simulink model "dynamic_twotrack_model"  (R2019a)
settings: Solver=VariableStepAuto  StartTime=0.0  StopTime=100  RelTol=1e-3
values from neighbouring files (symbols this model uses):
  cornering_stiffness = 1000    [config_dynamic_twotrack_model.m]
  init_states = [0; 0; 0; 0; 0; 0]    [config_dynamic_twotrack_model.m]
  length_front = 1    [config_dynamic_twotrack_model.m]
  length_rear = 1    [config_dynamic_twotrack_model.m]
  length_width = 0.5    [config_dynamic_twotrack_model.m]
  mass = 200    [config_dynamic_twotrack_model.m]
  yaw_inertia = 1000    [config_dynamic_twotrack_model.m]
libraries: simulink_extras x1, simulink x1
settings Model: Creator=jacoboffersen  LastModifiedBy=jacoboffersen

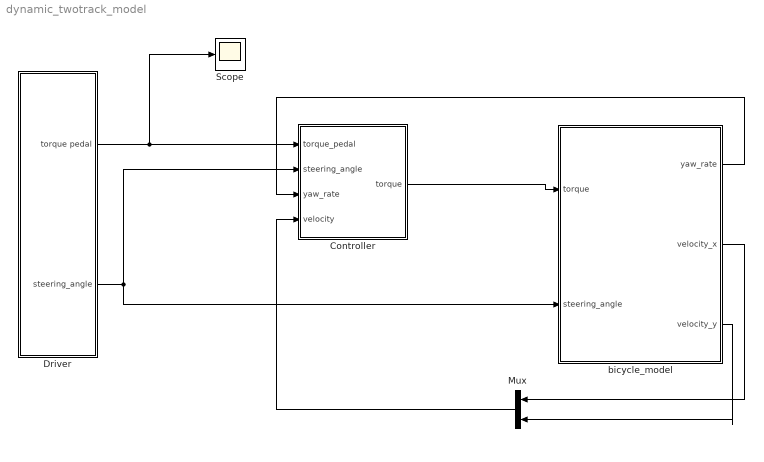
== system dynamic_twotrack_model ==
  Controller : Subsystem
  Driver : Subsystem
  Mux : Mux  Inputs=2
  Scope : Scope
  "bicycle_model " : Subsystem
  wires:
  Driver/2(steering_angle) -> "bicycle_model "/2("steering_angle "), Controller/2(steering_angle)
  Controller/1(torque) -> "bicycle_model "/1(torque)
  Driver/1(torque pedal) -> Scope/1, Controller/1(torque_pedal)
  Mux/1 -> Controller/4(velocity)
  "bicycle_model "/1(yaw_rate) -> Controller/3(yaw_rate)
  "bicycle_model "/2(velocity_x) -> Mux/1
  "bicycle_model "/3(velocity_y) -> Mux/2

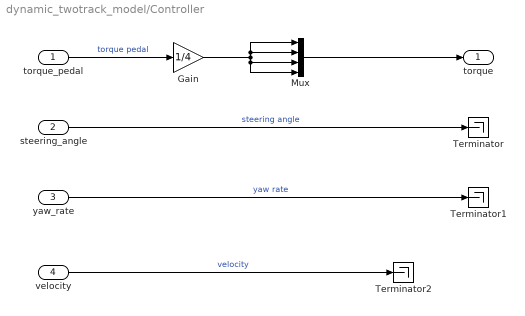
== system dynamic_twotrack_model/Controller ==
  torque_pedal : Inport
  steering_angle : Inport  Port=2
  yaw_rate : Inport  Port=3
  velocity : Inport  Port=4
  Gain : Gain  Gain=1/4
  Mux : Mux
  Terminator : Terminator
  Terminator1 : Terminator
  Terminator2 : Terminator
  torque : Outport
  wires:
  torque_pedal/1 -> Gain/1  "torque pedal"
  steering_angle/1 -> Terminator/1  "steering angle"
  yaw_rate/1 -> Terminator1/1  "yaw rate"
  velocity/1 -> Terminator2/1  "velocity"
  Mux/1 -> torque/1
  Gain/1 -> Mux/2, Mux/1, Mux/4, Mux/3

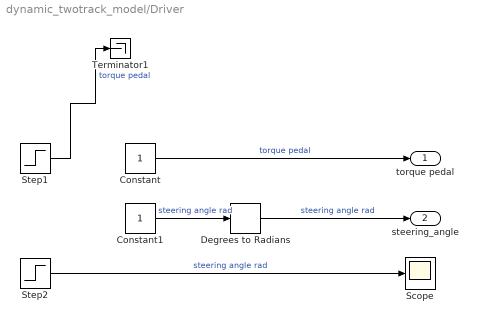
== system dynamic_twotrack_model/Driver ==
  Constant : Constant
  Constant1 : Constant
  Degrees to Radians : simulink_extras/Transformations/Degrees to Radians
  Scope : Scope
  Step1 : Step  Time=2  After=0  SampleTime=0
  Step2 : Step  Time=3  After=5  SampleTime=0
  Terminator1 : Terminator
  torque pedal : Outport
  steering_angle : Outport  Port=2
  wires:
  Constant/1 -> torque pedal/1  "torque pedal"
  Degrees to Radians/1 -> steering_angle/1  "steering angle rad"
  Step1/1 -> Terminator1/1  "torque pedal"
  Constant1/1 -> Degrees to Radians/1  "steering angle rad"
  Step2/1 -> Scope/1  "steering angle rad"

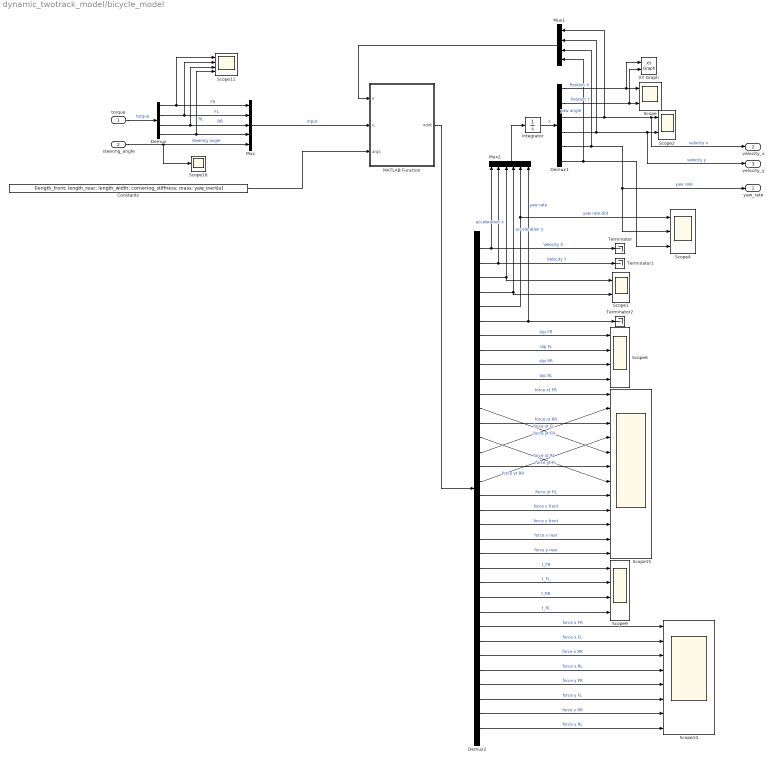
== system dynamic_twotrack_model/bicycle_model  ==
  torque : Inport
  "steering_angle " : Inport  Port=2
  Constants : Constant  Value=[length_front; length_rear; length_width; cornering_stiffness; mass; yaw_inertia]
  Demux : Demux
  Demux1 : Demux  Outputs=6
  Demux2 : Demux  Outputs=34
  Integrator : Integrator  InitialCondition=[init_states]
  MATLAB Function : MATLAB Function  TreatAsAtomicUnit=on
  Mux : Mux  Inputs=5
  Mux1 : Mux
  Mux2 : Mux  Inputs=6
  Scope : Scope  NumInputPorts=2
  Scope1 : Scope  NumInputPorts=2
  Scope10 : Scope
  Scope11 : Scope  NumInputPorts=4
  Scope14 : Scope  NumInputPorts=8
  Scope15 : Scope  NumInputPorts=12
  Scope2 : Scope  NumInputPorts=2
  Scope4 : Scope  NumInputPorts=3
  Scope6 : Scope  NumInputPorts=4
  Scope9 : Scope  NumInputPorts=4
  Terminator : Terminator
  Terminator1 : Terminator
  Terminator2 : Terminator
  XY Graph : simulink/Sinks/XY Graph  xmin=-10000  xmax=10000  ymin=-10000  ymax=10000  st=-1
  yaw_rate : Outport
  velocity_x : Outport  Port=2
  velocity_y : Outport  Port=3
  wires:
  Mux/1 -> MATLAB Function/2(u)  "input"
  "steering_angle "/1 -> Scope10/1, Mux/5  "steering angle"
  Constants/1 -> MATLAB Function/3(args)
  MATLAB Function/1(xdot) -> Demux2/1
  torque/1 -> Demux/1  "torque"
  Demux/4 -> Scope11/4, Mux/4  "RL"
  Demux/3 -> Scope11/3, Mux/3  "RR"
  Demux/2 -> Scope11/2, Mux/2  "FL"
  Demux/1 -> Scope11/1, Mux/1  "FR"
  Integrator/1 -> Demux1/1  "x"
  Mux1/1 -> MATLAB Function/1(x)
  Demux1/6 -> Scope4/3, Mux1/4  "yaw angle"
  Demux1/5 -> Mux1/3, Scope4/2, yaw_rate/1  "yaw rate"
  Demux1/4 -> velocity_y/1, Scope2/2, Mux1/2  "velocity y"
  Demux1/3 -> velocity_x/1, Scope2/1, Mux1/1  "velocity x"
  Demux2/1 -> Mux2/1, Terminator/1  "Velocity X"
  Demux2/2 -> Mux2/2, Terminator1/1  "Velocity Y"
  Demux2/3 -> Mux2/3, Scope1/1  "acceleration x"
  Demux2/4 -> Mux2/4, Scope1/2  "acceleration y"
  Demux2/5 -> Mux2/5, Scope4/1  "yaw rate dot"
  Demux2/6 -> Mux2/6, Terminator2/1  "yaw rate"
  Demux1/1 -> XY Graph/1, Scope/1  "Position X"
  Demux1/2 -> XY Graph/2, Scope/2  "Position Y"
  Mux2/1 -> Integrator/1
  Demux2/7 -> Scope6/1  "slip FR"
  Demux2/8 -> Scope6/2  "slip FL"
  Demux2/9 -> Scope6/3  "slip RR"
  Demux2/10 -> Scope6/4  "slip RL"
  Demux2/14 -> Scope15/7  "force xt RL"
  Demux2/13 -> Scope15/3  "force xt RR"
  Demux2/12 -> Scope15/5  "force xt FL"
  Demux2/11 -> Scope15/1  "force xt FR"
  Demux2/15 -> Scope15/2  "force yt FR"
  Demux2/16 -> Scope15/6  "force yt FL"
  Demux2/17 -> Scope15/4  "force yt RR"
  Demux2/18 -> Scope15/8  "force yt RL"
  Demux2/23 -> Scope9/1  "t_FR"
  Demux2/24 -> Scope9/2  "t_FL"
  Demux2/25 -> Scope9/3  "t_RR"
  Demux2/26 -> Scope9/4  "t_RL"
  Demux2/19 -> Scope15/9  "force x front"
  Demux2/20 -> Scope15/10  "force y front"
  Demux2/21 -> Scope15/11  "force x rear"
  Demux2/22 -> Scope15/12  "force y rear"
  Demux2/27 -> Scope14/1  "force x FR"
  Demux2/28 -> Scope14/2  "force x FL"
  Demux2/29 -> Scope14/3  "force x RR"
  Demux2/30 -> Scope14/4  "force x RL"
  Demux2/31 -> Scope14/5  "force y FR"
  Demux2/32 -> Scope14/6  "force y FL"
  Demux2/33 -> Scope14/7  "force y RR"
  Demux2/34 -> Scope14/8  "force y RL"

== matlab function dynamic_twotrack_model/bicycle_model /MATLAB Function ==
  data: x input; xdot output; u input; args input
function xdot = fcn(x, u, args)

% States
velocity_x       = x(1); 
velocity_y       = x(2); 
yaw_rate         = x(3); 
yaw_angle        = x(4); 

% System inputs
torque_FR        = u(1); 
torque_FL        = u(2); 
torque_RR        = u(3); 
torque_RL        = u(4); 
steering_angle   = u(5); 

% Constants
length_front        = args(1); 
length_rear         = args(2); 
length_width        = args(3); 
cornering_stiffness = args(4);
mass                = args(5);
yaw_inertia         = args(6);

g = 9.82;


Velocity_X = velocity_x * cos(yaw_angle) - velocity_y*sin(yaw_angle);
Velocity_Y = velocity_x * sin(yaw_angle) + velocity_y*cos(yaw_angle);


% Load transfer
lt_FR = 0;
lt_FL = 0;
lt_RR = 0;
lt_RL = 0;





% Vertical force on each wheel
force_z_FR = mass * g/4 + lt_FR;
force_z_FL = mass * g/4 + lt_FL;
force_z_RR = mass * g/4 + lt_RR;
force_z_RL = mass * g/4 + lt_RL;

% Longitudinal force on each wheel
force_x_factor = 1;
force_x_FR = torque_FR * force_z_FR * force_x_factor;
force_x_FL = torque_FL * force_z_FL * force_x_factor;
force_x_RR = torque_RR * force_z_RR * force_x_factor;
force_x_RL = torque_RL * force_z_RL * force_x_factor;


% Slip for each wheel
slip_FR = 0;
slip_FL = 0;
slip_RR = 0;
slip_RL = 0;
t_FR = 0;
t_FL = 0;
t_RR = 0;
t_RL = 0;
if velocity_x ~= 0 %&& yaw_rate ~= 0
%     slip_FR = steering_angle - atan((velocity_y+length_front*yaw_rate)/...
%                                     min(100000, velocity_x+length_width*yaw_rate));
% 
%     slip_FL = steering_angle - atan((velocity_y+length_front*yaw_rate)/...
%                                     min(100000, velocity_x-length_width*yaw_rate));
% 
%     slip_RR = - atan((velocity_y+length_rear*yaw_rate)/...
%                      min(100000, velocity_x+length_width*yaw_rate));
% 
%     slip_RL = - atan((velocity_y+length_rear*yaw_rate)/...
%                      min(100000, velocity_x-length_width*yaw_rate));
%     t_FR = - atan((velocity_y+length_front*yaw_rate)/...
%                   min(100000, velocity_x+length_width*yaw_rate));
%     t_FL = - atan((velocity_y+length_front*yaw_rate)/...
%                   min(100000, velocity_x-length_width*yaw_rate));
%     t_RR = - atan((velocity_y+length_rear*yaw_rate)/...
%                   min(100000, velocity_x+length_width*yaw_rate));
%     t_RL = - atan((velocity_y+length_rear*yaw_rate)/...
%                   min(100000, velocity_x-length_width*yaw_rate));
end
% 
slip_FR =   steering_angle * velocity_x * 0.1;
slip_FL =   steering_angle * velocity_x * 0.1;
slip_RR = - steering_angle * velocity_x * 0.05;
slip_RL = - steering_angle * velocity_x * 0.05;


% if velocity_x ~= 0 %&& yaw_rate ~= 0
%     beta = atan(length_rear/(length_front+length_rear)*tan(steering_angle));
%     slip_FR = steering_angle - beta - 1/velocity_x*(length_front/length_width)*yaw_rate;
%     slip_FL = steering_angle - beta - 1/velocity_x*(length_front/(length_width))*yaw_rate;
%     slip_RR = - atan((velocity_y+length_rear*yaw_rate)/...
%                      (velocity_x+length_width*yaw_rate));
% 
%     slip_RL = - atan((velocity_y+length_rear*yaw_rate)/...
%                      (velocity_x-length_width*yaw_rate));
% end

% Lateral force on each wheel
force_y_FR = cornering_stiffness * slip_FR;
force_y_FL = cornering_stiffness * slip_FL;
force_y_RR = cornering_stiffness * slip_RR;
force_y_RL = cornering_stiffness * slip_RL;

% Each force composant on each wheel
% FR
F_xx_FR = force_x_FR*cos(steering_angle);
F_xy_FR = force_x_FR*sin(steering_angle);
F_yy_FR = force_y_FR*cos(steering_angle);
F_yx_FR = force_y_FR*sin(steering_angle);


% FL
F_xx_FL = force_x_FL*cos(steering_angle);
F_xy_FL = force_x_FL*sin(steering_angle);
F_yy_FL = force_y_FL*cos(steering_angle);
F_yx_FL = force_y_FL*sin(steering_angle);

% RL
F_x_RL = force_x_RL;
F_y_RL = force_y_RL;

% RR
F_x_RR = force_x_RR;
F_y_RR = force_y_RR;

% Actual forces on each wheel in x and y directions
force_xt_FR = F_xx_FR - F_yx_FR;
force_xt_FL = F_yx_FL - F_xx_FL;
force_xt_RR = F_x_RR;
force_xt_RL = F_x_RL;

force_yt_FR = F_xy_FR + F_yy_FR;
force_yt_FL = F_xy_FL + F_yy_FL;
force_yt_RR = F_y_RR;
force_yt_RL = F_y_RL;

% Combined forces
force_x_front = force_xt_FR + force_xt_FL; 
force_y_front = force_yt_FR + force_yt_FL; 
force_x_rear  = force_xt_RR + force_xt_RL;
force_y_rear  = force_yt_RR + force_yt_RL;

force_fric = 1; %velocity_x * 1.5;
% force_fric = velocity_x * 100;
acceleration_x =  yaw_rate*velocity_y + 1/mass*(force_x_front + force_x_rear)-force_fric;

acceleration_y = -yaw_rate*velocity_x + 1/mass*(force_y_front + force_y_rear);



% Yaw rate dot
yaw_rate_dot = 1/yaw_inertia * (force_y_front*length_front - ...
                                force_y_rear*length_rear + ...
                                (force_x_front - force_x_rear)*length_width);
                            
% yaw_rate_dot = 1/yaw_inertia*(length_front*(force_y_FR+force_y_FL)-...
%                               length_rear *(force_y_RR+force_y_RL)+...
%                               length_width*(force_x_FR+force_x_RR-force_x_FL-force_x_RL));

xdot = [Velocity_X; Velocity_Y; acceleration_x; acceleration_y; yaw_rate_dot; yaw_rate;
        slip_FR; slip_FL; slip_RR; slip_RL;
        force_xt_FR; force_xt_FL ; force_xt_RR; force_xt_RL;
        force_yt_FR; force_yt_FL ; force_yt_RR; force_yt_RL;
        force_x_front; force_y_front ; force_x_rear; force_y_rear;
        t_FR; t_FL; t_RR; t_RL;
        force_x_FR; force_x_FL ; force_x_RR; force_x_RL;
        force_y_FR; force_y_FL ; force_y_RR; force_y_RL];
